simulink model "SolarPoweredPMSMDrive"  (R2024b)
settings: Solver=VariableStepAuto  StartTime=0.0  StopTime=1.5  RelTol=1e-3
libraries: spsSeriesRLCBranchLib x8, spsIGBTDiodeLib x7, spsVoltageMeasurementLib x4, spsCurrentMeasurementLib x1, spsDiodeLib x1, spsGroundLib x1, spsPVArrayLib x1, spsPWMGeneratorDCDCLib x1, simulink x1, sps_lib x1
settings Model: Creator=ASUS  LastModifiedBy=ASUS

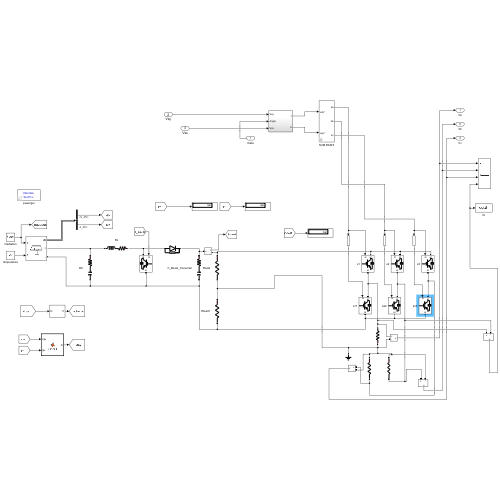
[thumbnail: Simulink's stored preview of the top-level diagram]
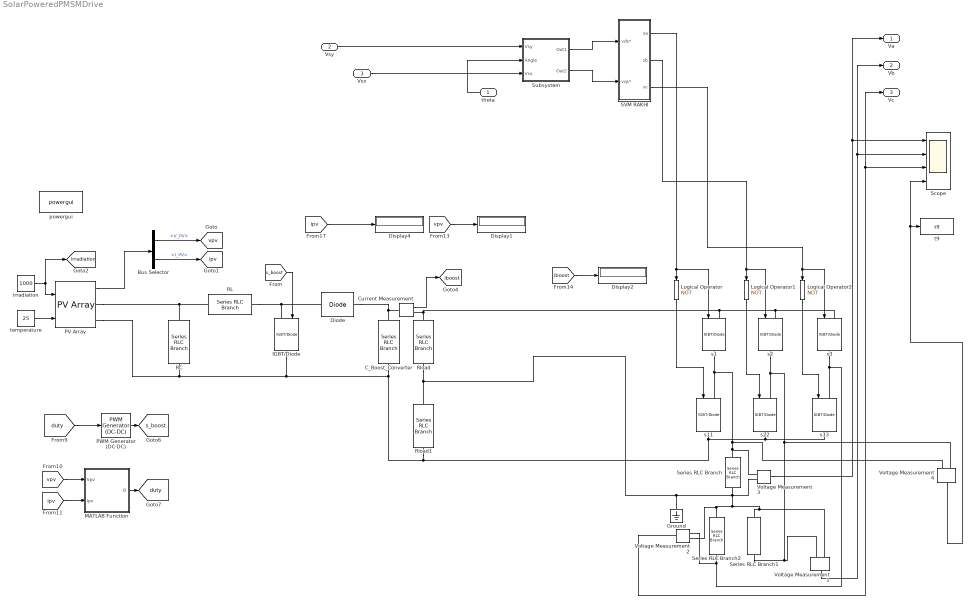
== system SolarPoweredPMSMDrive ==
  theta : Inport
  Vsy : Inport  Port=2
  Vsx : Inport  Port=3
  Bus Selector : BusSelector  OutputSignals=V_PV,I_PV
  C_Boost_Converter : spsSeriesRLCBranchLib/Series RLC Branch  LConnTagsString=__new0  RConnTagsString=__new0  BranchType=RC  Resistance=1e-4  Inductance=1e-3  SetiL0=off  InitialCurrent=0  Capacitance=660e-5  Setx0=off  InitialVoltage=0  Measurements=None
  Current Measurement : spsCurrentMeasurementLib/Current Measurement  PhasorSimulation=off  OutputType=Complex  PSBequivalent=0
  Diode : spsDiodeLib/Diode  Ron=0.001  Lon=0  Vf=0.8  IC=0  UseSnubber=0  Rs=500  Cs=250e-9  Measurements=off
  Display1 : Display
  Display2 : Display
  Display4 : Display
  Ground : spsGroundLib/Ground  LConnTagsString=a
  IGBT/Diode : spsIGBTDiodeLib/IGBT//Diode  Ron=1e-3  Rs=1e5  Cs=inf  Measurements=off
  Logical Operator : Logic  Operator=NOT  AllPortsSameDT=off  OutDataTypeStr=boolean
  Logical Operator1 : Logic  Operator=NOT  AllPortsSameDT=off  OutDataTypeStr=boolean
  Logical Operator2 : Logic  Operator=NOT  AllPortsSameDT=off  OutDataTypeStr=boolean
  MATLAB Function : MATLAB Function  TreatAsAtomicUnit=on
  PV Array : spsPVArrayLib/PV Array  Npar=10  Nser=10  PlotType=array @ 1000 W/m2 & specified temperatures  S_vec="[ 1000  500  100 ]"  Temp_C_vec="[ 45 25  ]"  ModuleName=User-defined  PlotWhenSelected=off  Pm=213.15  Ncell=60  Voc=36.3  Isc=7.84  Vm=29  Im=7.35  beta_Voc_pc=-0.36099  alpha_Isc_pc=0.102  beta_Voc=-0.13104  alpha_Isc=0.0079968  IL=7.8654  I0=2.9273e-10  nI=0.98119  Rsh=313.0553  Rs=0.39381  RobustModel=off  RobustCellTemperature=313.3991  BAL=on  Tc=1e-6  Tfilter=5e-5
  PWM Generator (DC-DC) : spsPWMGeneratorDCDCLib/PWM Generator (DC-DC)  Fsw=5000  Ts=10e-6
  RC : spsSeriesRLCBranchLib/Series RLC Branch  LConnTagsString=__new0  RConnTagsString=__new0  BranchType=RC  Resistance=1e-4  Inductance=1e-3  SetiL0=off  InitialCurrent=0  Capacitance=20e-6  Setx0=off  InitialVoltage=0  Measurements=None
  RL : spsSeriesRLCBranchLib/Series RLC Branch  LConnTagsString=__new0  RConnTagsString=__new0  BranchType=RL  Resistance=0.1  Inductance=1e-3  SetiL0=off  InitialCurrent=0  Capacitance=1e-6  Setx0=off  InitialVoltage=0  Measurements=None
  Rload : spsSeriesRLCBranchLib/Series RLC Branch  LConnTagsString=__new0  RConnTagsString=__new0  BranchType=R  Resistance=5  Inductance=1e-3  SetiL0=off  InitialCurrent=0  Capacitance=1e-6  Setx0=off  InitialVoltage=0  Measurements=None
  Rload1 : spsSeriesRLCBranchLib/Series RLC Branch  LConnTagsString=__new0  RConnTagsString=__new0  BranchType=R  Resistance=5  Inductance=1e-3  SetiL0=off  InitialCurrent=0  Capacitance=1e-6  Setx0=off  InitialVoltage=0  Measurements=None
  SVM RAKHI : Subsystem  mask{Ts=200e-6, Vdc=400}
  Scope : Scope  NumInputPorts=4
  Series RLC Branch : spsSeriesRLCBranchLib/Series RLC Branch  LConnTagsString=__new0  RConnTagsString=__new0  BranchType=R  Resistance=2  Inductance=3e-3  SetiL0=off  InitialCurrent=0  Capacitance=1e-6  Setx0=off  InitialVoltage=0  Measurements=None
  Series RLC Branch1 : spsSeriesRLCBranchLib/Series RLC Branch  LConnTagsString=__new0  RConnTagsString=__new0  BranchType=R  Resistance=2  Inductance=3e-3  SetiL0=off  InitialCurrent=0  Capacitance=1e-6  Setx0=off  InitialVoltage=0  Measurements=None
  Series RLC Branch2 : spsSeriesRLCBranchLib/Series RLC Branch  LConnTagsString=__new0  RConnTagsString=__new0  BranchType=R  Resistance=2  Inductance=3e-3  SetiL0=off  InitialCurrent=0  Capacitance=1e-6  Setx0=off  InitialVoltage=0  Measurements=None
  Subsystem : Subsystem
  Voltage Measurement{1..4} (4 alike) : spsVoltageMeasurementLib/Voltage Measurement  PhasorSimulation=off  OutputType=Complex  PSBequivalent=0
  irradiation : Constant  Value=1000
  powergui : sps_lib/powergui  Priority=1  SimulationMode=Discrete  SampleTime=50e-6  frequency=60  Iterations=50  frequencyindice=0  Pbase=100e6  ErrMax=1e-4  UnitsV=kV  UnitsW=MW  buscounter=0  FunctionMessages=off  echomessages=off  EnableUseOfTLC=off  CurrentSourceSwitches=off  DisableSnubberDevices=off  DisableRonSwitches=off  DisableVfSwitches=off  DisplayEquations=off  AutomaticDiscreteSolvers=off  SolverType=Tustin/Backward Euler (TBE)  Interpol=off  ExternalGateDelay=off  methode=off  Ts=100  x0status=blocks  SPID=on  SwTol=0  HookPort=off  NonlinearTolerance=1e-4  nMaxIteration=100  ContinueOnMaxIteration=off  RestoreLinks=warning  ResistiveCurrentMeasurement=off  Frange=[0:2:500]  Ylog=off  Xlog=on  ShowGrid=off  save=off  variable=ZData  structure=0  ZoomFFT=off  StartTime=0.0  cycles=1  DisplayStyle=1  fundamental=60  FreqAxis=off  MaxFrequency=1000  frequencyindicesteady=1  RmsSteady=1  display=off
  s{1..3,11,22,33} (6 alike) : spsIGBTDiodeLib/IGBT//Diode  Ron=1e-3  Rs=1e5  Cs=inf  Measurements=off
  t9 : ToWorkspace  VariableName=t9  SaveFormat=Structure With Time  SampleTime=-1
  temperature : Constant  Value=25
  Va : Outport
  Vb : Outport  Port=2
  Vc : Outport  Port=3
  tag scope: duty=global, iboost=global, ipv=global, irradiation=global, s_boost=global, vpv=global
  wires:
  Voltage Measurement3/1 -> Va/1, Scope/1
  Logical Operator2/1 -> s33/1
  Subsystem/1(Out1) -> SVM RAKHI/1(vds*)
  Bus Selector/1 -> [vpv]  "<V_PV>"
  irradiation/1 -> PV Array/1, [irradiation]
  [duty] -> PWM Generator (DC-DC)/1
  Bus Selector/2 -> [ipv]  "<I_PV>"
  theta/1 -> Subsystem/2(Angle)
  Voltage Measurement1/1 -> Vb/1, Scope/2
  PWM Generator (DC-DC)/1 -> [s_boost]
  [s_boost] -> IGBT/Diode/1
  [iboost] -> Display2/1
  Voltage Measurement4/1 -> t9/1, Scope/4
  [ipv] -> MATLAB Function/2(Ipv)
  SVM RAKHI/2(sb) -> Logical Operator1/1, s2/1
  [vpv] -> MATLAB Function/1(Vpv)
  Voltage Measurement2/1 -> Scope/3, Vc/1
  SVM RAKHI/3(sc) -> Logical Operator2/1, s3/1
  Vsx/1 -> Subsystem/3(Vsx)
  [vpv] -> Display1/1
  PV Array/1 -> Bus Selector/1
  Current Measurement/1 -> [iboost]
  Subsystem/2(Out2) -> SVM RAKHI/2(vqs*)
  temperature/1 -> PV Array/2
  MATLAB Function/1(D) -> [duty]
  Vsy/1 -> Subsystem/1(Vsy)
  [ipv] -> Display4/1
  Logical Operator/1 -> s11/1
  Logical Operator1/1 -> s22/1
  SVM RAKHI/1(sa) -> Logical Operator/1, s1/1
  connections:
  Diode/RConn1 -- Current Measurement/LConn1 -- C_Boost_Converter/LConn1
  Series RLC Branch1/RConn1 -- Voltage Measurement1/LConn1 -- s22/LConn1 -- s2/RConn1 -- Voltage Measurement4/LConn2
  PV Array/RConn1 -- RL/RConn1 -- RC/LConn1
  s1/RConn1 -- Voltage Measurement3/LConn1 -- Series RLC Branch/RConn1 -- Voltage Measurement4/LConn1 -- s11/LConn1
  s3/RConn1 -- Voltage Measurement2/LConn1 -- Series RLC Branch2/RConn1 -- s33/LConn1
  s22/RConn1 -- s33/RConn1 -- s11/RConn1 -- Rload1/RConn1 -- C_Boost_Converter/RConn1 -- IGBT/Diode/RConn1 -- PV Array/RConn2 -- RC/RConn1
  Voltage Measurement2/LConn2 -- Series RLC Branch2/LConn1 -- Series RLC Branch1/LConn1 -- Voltage Measurement1/LConn2 -- Voltage Measurement3/LConn2 -- Ground/LConn1 -- Rload1/LConn1 -- Rload/RConn1 -- Series RLC Branch/LConn1
  s2/LConn1 -- Rload/LConn1 -- Current Measurement/RConn1 -- s1/LConn1 -- s3/LConn1
  Diode/LConn1 -- RL/LConn1 -- IGBT/Diode/LConn1

== system SolarPoweredPMSMDrive/SVM RAKHI ==
  vds* : Inport
  vqs* : Inport  Port=2
  Angle Estimator : Subsystem  mask(angle estimator){}
  twolevel svm1rakhi : Subsystem
  sa : Outport
  sb : Outport  Port=2
  sc : Outport  Port=3
  wires:
  vqs*/1 -> Angle Estimator/2(vqs*)
  vds*/1 -> Angle Estimator/1(vds*)
  Angle Estimator/1(alpha) -> twolevel svm1rakhi/1(alpha)
  Angle Estimator/2(vref) -> twolevel svm1rakhi/2(VS)
  twolevel svm1rakhi/1(Sa) -> sa/1
  twolevel svm1rakhi/2(Sb) -> sb/1
  twolevel svm1rakhi/3(Sc) -> sc/1

== system SolarPoweredPMSMDrive/Subsystem ==
  Vsy : Inport
  Angle : Inport  Port=2
  Vsx : Inport  Port=3
  Mux1 : Mux  Inputs=3
      settings: DisplayOption=signals
  Vds : Fcn  Expr=(cos(u(3))*u(1))-(sin(u(3))*u(2))
  Vqs : Fcn  Expr=(cos(u(3))*u(2))+(sin(u(3))*u(1))
  Out1 : Outport
  Out2 : Outport  Port=2
  wires:
  Vds/1 -> Out1/1
  Vsy/1 -> Mux1/2
  Vsx/1 -> Mux1/1
  Angle/1 -> Mux1/3
  Vqs/1 -> Out2/1
  Mux1/1 -> Vds/1, Vqs/1

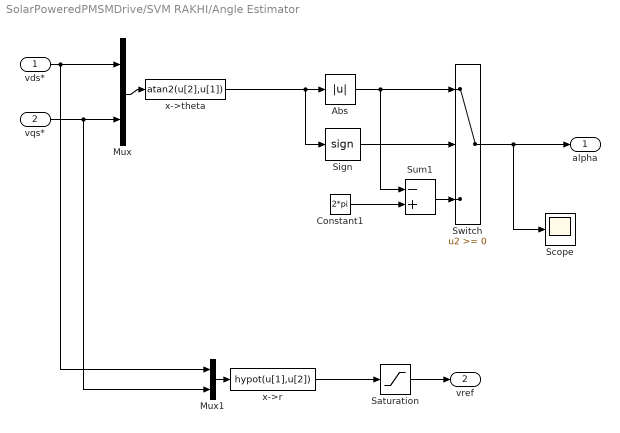
== system SolarPoweredPMSMDrive/SVM RAKHI/Angle Estimator ==
  vds* : Inport
  vqs* : Inport  Port=2
  Abs : Abs
  Constant1 : Constant  Value=2*pi
  Mux : Mux  Inputs=2
  Mux1 : Mux  Inputs=2
  Saturation : Saturate  UpperLimit=Vdc/1.732  LowerLimit=0
  Scope : Scope
  Sign : Signum
  Sum1 : Sum  Inputs=-+  InputSameDT=on  SaturateOnIntegerOverflow=on  OutDataTypeStr=Inherit: Same as first input
  Switch : Switch
  x->r : Fcn  Expr=hypot(u[1],u[2])
  x->theta : Fcn  Expr=atan2(u[2],u[1])
  alpha : Outport
  vref : Outport  Port=2
  wires:
  Abs/1 -> Sum1/1, Switch/1
  Sign/1 -> Switch/2
  Constant1/1 -> Sum1/2
  Sum1/1 -> Switch/3
  Switch/1 -> Scope/1, alpha/1
  x->theta/1 -> Sign/1, Abs/1
  Mux/1 -> x->theta/1
  x->r/1 -> Saturation/1
  vqs*/1 -> Mux/2, Mux1/2
  vds*/1 -> Mux/1, Mux1/1
  Mux1/1 -> x->r/1
  Saturation/1 -> vref/1

== system SolarPoweredPMSMDrive/SVM RAKHI/twolevel svm1rakhi ==
  alpha : Inport
  VS : Inport  Port=2
  Repeating Sequence : simulink/Sources/Repeating Sequence  rep_seq_t=[0 200e-6]  rep_seq_y=[0 200e-6]
  Subsystem2 : Subsystem
  Subsystem3 : Subsystem  mask{Ts=200e-6, Vdc=530}
  final two level pulses : Subsystem
  Sa : Outport
  Sb : Outport  Port=2
  Sc : Outport  Port=3
  wires:
  Subsystem3/2(Tb) -> final two level pulses/4(Tb)
  Subsystem3/3(T0) -> final two level pulses/5(T0)
  Repeating Sequence/1 -> final two level pulses/2(Cr)
  Subsystem3/1(Ta) -> final two level pulses/3(Ta)
  Subsystem2/1(K) -> Subsystem3/1(K), final two level pulses/1(K)
  alpha/1 -> Subsystem2/1(alpha), Subsystem3/2(ALPHA)
  VS/1 -> Subsystem3/3(VS)
  final two level pulses/2(Sb) -> Sb/1
  final two level pulses/1(Sa) -> Sa/1
  final two level pulses/3(Sc) -> Sc/1

== system SolarPoweredPMSMDrive/SVM RAKHI/twolevel svm1rakhi/Subsystem2 ==
  alpha : Inport
  Display : Display
  Fcn : Fcn  Expr=(3*u/pi)+1
  Rounding Function : Rounding  Operator=fix
  K : Outport
  wires:
  Fcn/1 -> Rounding Function/1
  alpha/1 -> Fcn/1
  Rounding Function/1 -> K/1, Display/1

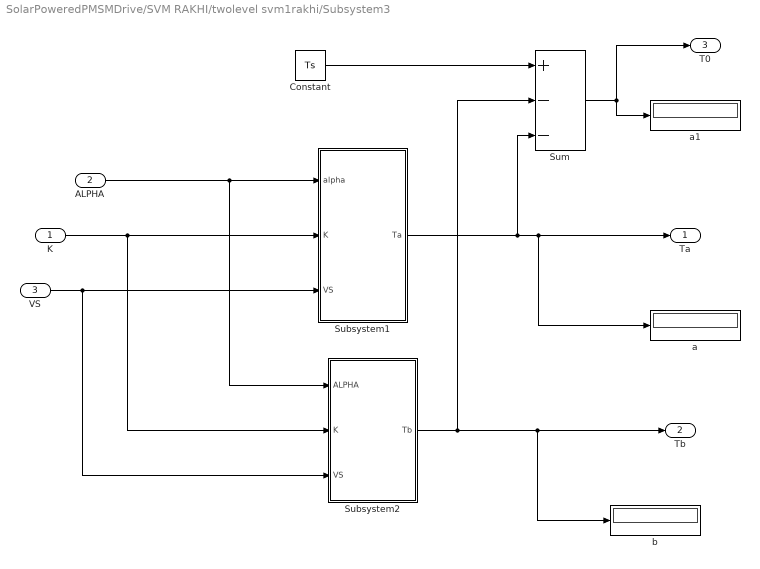
== system SolarPoweredPMSMDrive/SVM RAKHI/twolevel svm1rakhi/Subsystem3 ==
  K : Inport
  ALPHA : Inport  Port=2
  VS : Inport  Port=3
  Constant : Constant  Value=Ts
  Subsystem1 : Subsystem
  Subsystem2 : Subsystem
  Sum : Sum  Inputs=+--
  a : Display
  a1 : Display
  b : Display
  Ta : Outport
  Tb : Outport  Port=2
  T0 : Outport  Port=3
  wires:
  Sum/1 -> a1/1, T0/1
  Constant/1 -> Sum/1
  Subsystem2/1(Tb) -> b/1, Tb/1, Sum/2
  K/1 -> Subsystem2/2(K), Subsystem1/2(K)
  Subsystem1/1(Ta) -> a/1, Ta/1, Sum/3
  ALPHA/1 -> Subsystem1/1(alpha), Subsystem2/1(ALPHA)
  VS/1 -> Subsystem1/3(VS), Subsystem2/3(VS)

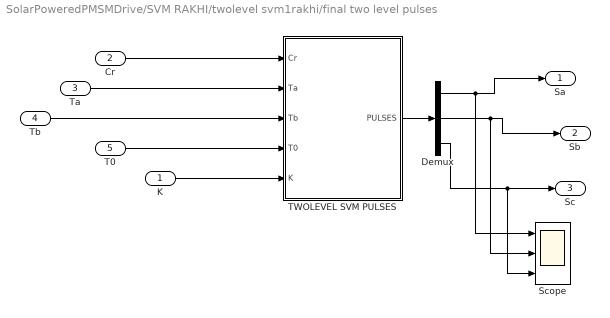
== system SolarPoweredPMSMDrive/SVM RAKHI/twolevel svm1rakhi/final two level pulses ==
  K : Inport
  Cr : Inport  Port=2
  Ta : Inport  Port=3
  Tb : Inport  Port=4
  T0 : Inport  Port=5
  Demux : Demux  Outputs=3
  Scope : Scope  NumInputPorts=3
  TWOLEVEL SVM PULSES : Subsystem
  Sa : Outport
  Sb : Outport  Port=2
  Sc : Outport  Port=3
  wires:
  TWOLEVEL SVM PULSES/1(PULSES) -> Demux/1
  Cr/1 -> TWOLEVEL SVM PULSES/1(Cr)
  Ta/1 -> TWOLEVEL SVM PULSES/2(Ta)
  Demux/3 -> Sc/1, Scope/3
  T0/1 -> TWOLEVEL SVM PULSES/4(T0)
  Demux/1 -> Sa/1, Scope/1
  Tb/1 -> TWOLEVEL SVM PULSES/3(Tb)
  Demux/2 -> Sb/1, Scope/2
  K/1 -> TWOLEVEL SVM PULSES/5(K)

== system SolarPoweredPMSMDrive/SVM RAKHI/twolevel svm1rakhi/Subsystem3/Subsystem1 ==
  alpha : Inport
  K : Inport  Port=2
  VS : Inport  Port=3
  Display : Display
  Fcn : Fcn  Expr=sin(u)
  Gain : Gain  Gain=pi/3
  Gain1 : Gain  Gain=(Ts/Vdc)*1.732
  Product1 : Product
  Sum : Sum  Inputs=-+
  Ta : Outport
  wires:
  alpha/1 -> Sum/1
  Product1/1 -> Ta/1, Display/1
  Sum/1 -> Fcn/1
  Gain/1 -> Sum/2
  Fcn/1 -> Gain1/1
  Gain1/1 -> Product1/1
  K/1 -> Gain/1
  VS/1 -> Product1/2

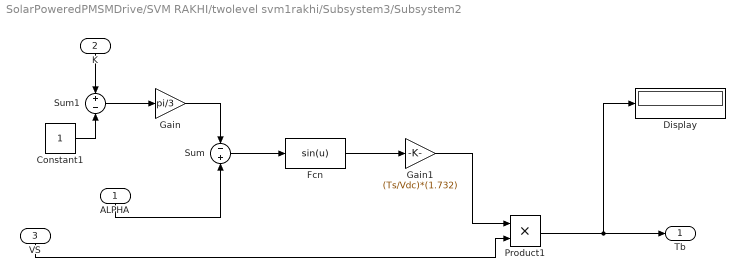
== system SolarPoweredPMSMDrive/SVM RAKHI/twolevel svm1rakhi/Subsystem3/Subsystem2 ==
  ALPHA : Inport
  K : Inport  Port=2
  VS : Inport  Port=3
  Constant1 : Constant
  Display : Display
  Fcn : Fcn  Expr=sin(u)
  Gain : Gain  Gain=pi/3
  Gain1 : Gain  Gain=(Ts/Vdc)*(1.732)
  Product1 : Product
  Sum : Sum  Inputs=-+
  Sum1 : Sum  Inputs=+-
  Tb : Outport
  wires:
  Sum/1 -> Fcn/1
  Fcn/1 -> Gain1/1
  Gain/1 -> Sum/1
  Gain1/1 -> Product1/1
  K/1 -> Sum1/1
  ALPHA/1 -> Sum/2
  VS/1 -> Product1/2
  Constant1/1 -> Sum1/2
  Product1/1 -> Tb/1, Display/1
  Sum1/1 -> Gain/1

== system SolarPoweredPMSMDrive/SVM RAKHI/twolevel svm1rakhi/final two level pulses/TWOLEVEL SVM PULSES ==
  Cr : Inport
  Ta : Inport  Port=2
  Tb : Inport  Port=3
  T0 : Inport  Port=4
  K : Inport  Port=5
  Multiport Switch : MultiPortSwitch  Inputs=6  DiagnosticForDefault=None  SaturateOnIntegerOverflow=off  InputSameDT=off
  PULSES FOR ALL SECTORS : Subsystem
  PULSES : Outport
  wires:
  K/1 -> Multiport Switch/1
  Ta/1 -> PULSES FOR ALL SECTORS/2(Ta)
  Tb/1 -> PULSES FOR ALL SECTORS/3(Tb)
  T0/1 -> PULSES FOR ALL SECTORS/4(T0)
  PULSES FOR ALL SECTORS/2(sector2) -> Multiport Switch/3
  PULSES FOR ALL SECTORS/1(sector1) -> Multiport Switch/2
  PULSES FOR ALL SECTORS/5(sector5) -> Multiport Switch/6
  PULSES FOR ALL SECTORS/4(sector4) -> Multiport Switch/5
  PULSES FOR ALL SECTORS/3(sector3) -> Multiport Switch/4
  PULSES FOR ALL SECTORS/6(sector6) -> Multiport Switch/7
  Cr/1 -> PULSES FOR ALL SECTORS/1(Cr)
  Multiport Switch/1 -> PULSES/1

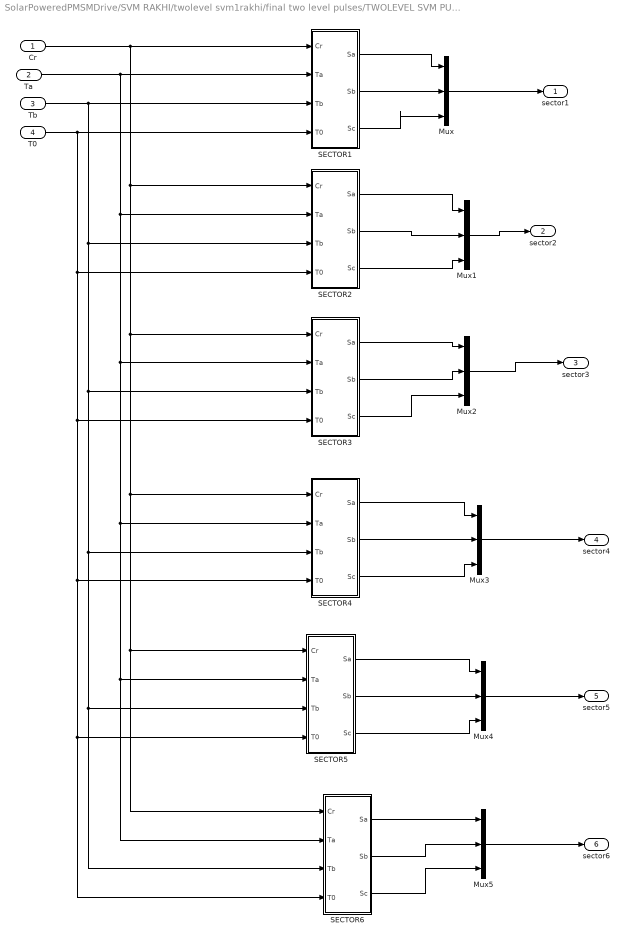
== system SolarPoweredPMSMDrive/SVM RAKHI/twolevel svm1rakhi/final two level pulses/TWOLEVEL SVM PULSES/PULSES FOR ALL SECTORS ==
  Cr : Inport
  Ta : Inport  Port=2
  Tb : Inport  Port=3
  T0 : Inport  Port=4
  Mux{,1..5} (6 alike) : Mux  Inputs=3
  SECTOR1 : Subsystem
  SECTOR2 : Subsystem
  SECTOR3 : Subsystem
  SECTOR4 : Subsystem
  SECTOR5 : Subsystem
  SECTOR6 : Subsystem
  sector1 : Outport
  sector2 : Outport  Port=2
  sector3 : Outport  Port=3
  sector4 : Outport  Port=4
  sector5 : Outport  Port=5
  sector6 : Outport  Port=6
  wires:
  SECTOR6/3(Sc) -> Mux5/3
  Mux4/1 -> sector5/1
  Mux/1 -> sector1/1
  Mux5/1 -> sector6/1
  Mux3/1 -> sector4/1
  SECTOR6/2(Sb) -> Mux5/2
  SECTOR5/3(Sc) -> Mux4/3
  Mux1/1 -> sector2/1
  SECTOR5/2(Sb) -> Mux4/2
  Mux2/1 -> sector3/1
  SECTOR3/2(Sb) -> Mux2/2
  SECTOR1/1(Sa) -> Mux/1
  SECTOR1/2(Sb) -> Mux/2
  SECTOR4/2(Sb) -> Mux3/2
  SECTOR4/3(Sc) -> Mux3/3
  SECTOR2/1(Sa) -> Mux1/1
  SECTOR6/1(Sa) -> Mux5/1
  SECTOR1/3(Sc) -> Mux/3
  SECTOR3/1(Sa) -> Mux2/1
  SECTOR4/1(Sa) -> Mux3/1
  SECTOR3/3(Sc) -> Mux2/3
  SECTOR5/1(Sa) -> Mux4/1
  SECTOR2/3(Sc) -> Mux1/3
  SECTOR2/2(Sb) -> Mux1/2
  Cr/1 -> SECTOR1/1(Cr), SECTOR2/1(Cr), SECTOR4/1(Cr), SECTOR6/1(Cr), SECTOR5/1(Cr), SECTOR3/1(Cr)
  T0/1 -> SECTOR6/4(T0), SECTOR5/4(T0), SECTOR4/4(T0), SECTOR3/4(T0), SECTOR2/4(T0), SECTOR1/4(T0)
  Ta/1 -> SECTOR1/2(Ta), SECTOR3/2(Ta), SECTOR4/2(Ta), SECTOR6/2(Ta), SECTOR5/2(Ta), SECTOR2/2(Ta)
  Tb/1 -> SECTOR1/3(Tb), SECTOR5/3(Tb), SECTOR6/3(Tb), SECTOR4/3(Tb), SECTOR3/3(Tb), SECTOR2/3(Tb)

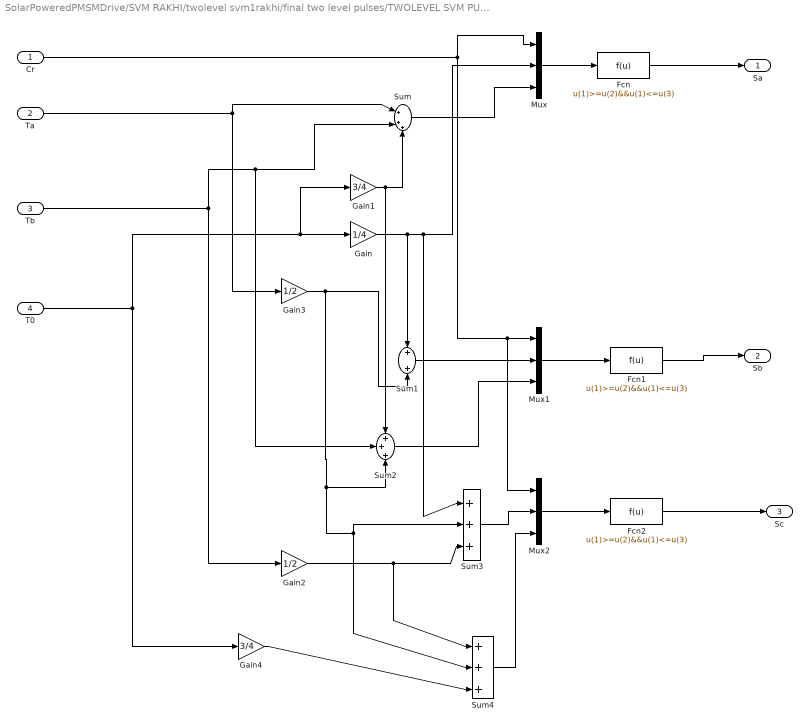
== system SolarPoweredPMSMDrive/SVM RAKHI/twolevel svm1rakhi/final two level pulses/TWOLEVEL SVM PULSES/PULSES FOR ALL SECTORS/SECTOR1 ==
  Cr : Inport
  Ta : Inport  Port=2
  Tb : Inport  Port=3
  T0 : Inport  Port=4
  Fcn : Fcn  Expr=u(1)>=u(2)&&u(1)<=u(3)
  Fcn1 : Fcn  Expr=u(1)>=u(2)&&u(1)<=u(3)
  Fcn2 : Fcn  Expr=u(1)>=u(2)&&u(1)<=u(3)
  Gain : Gain  Gain=1/4
  Gain1 : Gain  Gain=3/4
  Gain2 : Gain  Gain=1/2
  Gain3 : Gain  Gain=1/2
  Gain4 : Gain  Gain=3/4
  Mux : Mux  Inputs=3
  Mux1 : Mux  Inputs=3
  Mux2 : Mux  Inputs=3
  Sum : Sum  Inputs=|+++
  Sum1 : Sum
  Sum2 : Sum  Inputs=+++
  Sum3 : Sum  Inputs=|+++
  Sum4 : Sum  Inputs=|+++
  Sa : Outport
  Sb : Outport  Port=2
  Sc : Outport  Port=3
  wires:
  Sum2/1 -> Mux1/3
  Mux/1 -> Fcn/1
  T0/1 -> Gain4/1, Gain1/1, Gain/1
  Sum1/1 -> Mux1/2
  Mux2/1 -> Fcn2/1
  Gain3/1 -> Sum4/2, Sum3/2, Sum2/3, Sum1/2
  Gain1/1 -> Sum/3, Sum2/1
  Sum/1 -> Mux/3
  Fcn2/1 -> Sc/1
  Sum4/1 -> Mux2/3
  Cr/1 -> Mux/1, Mux2/1, Mux1/1
  Fcn/1 -> Sa/1
  Gain2/1 -> Sum4/1, Sum3/3
  Mux1/1 -> Fcn1/1
  Sum3/1 -> Mux2/2
  Gain4/1 -> Sum4/3
  Fcn1/1 -> Sb/1
  Gain/1 -> Sum3/1, Mux/2, Sum1/1
  Ta/1 -> Gain3/1, Sum/1
  Tb/1 -> Sum2/2, Sum/2, Gain2/1

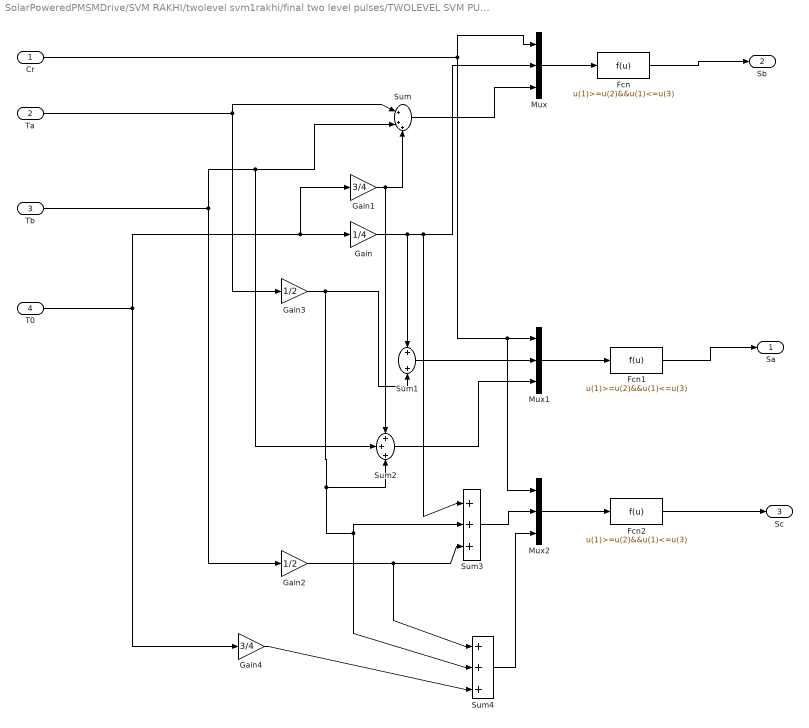
== system SolarPoweredPMSMDrive/SVM RAKHI/twolevel svm1rakhi/final two level pulses/TWOLEVEL SVM PULSES/PULSES FOR ALL SECTORS/SECTOR2 ==
  Cr : Inport
  Ta : Inport  Port=2
  Tb : Inport  Port=3
  T0 : Inport  Port=4
  Fcn : Fcn  Expr=u(1)>=u(2)&&u(1)<=u(3)
  Fcn1 : Fcn  Expr=u(1)>=u(2)&&u(1)<=u(3)
  Fcn2 : Fcn  Expr=u(1)>=u(2)&&u(1)<=u(3)
  Gain : Gain  Gain=1/4
  Gain1 : Gain  Gain=3/4
  Gain2 : Gain  Gain=1/2
  Gain3 : Gain  Gain=1/2
  Gain4 : Gain  Gain=3/4
  Mux : Mux  Inputs=3
  Mux1 : Mux  Inputs=3
  Mux2 : Mux  Inputs=3
  Sum : Sum  Inputs=|+++
  Sum1 : Sum
  Sum2 : Sum  Inputs=+++
  Sum3 : Sum  Inputs=|+++
  Sum4 : Sum  Inputs=|+++
  Sa : Outport
  Sb : Outport  Port=2
  Sc : Outport  Port=3
  wires:
  Fcn2/1 -> Sc/1
  Fcn/1 -> Sb/1
  Fcn1/1 -> Sa/1
  Tb/1 -> Gain2/1, Sum/2, Sum2/2
  Ta/1 -> Sum/1, Gain3/1
  Gain/1 -> Sum1/1, Mux/2, Sum3/1
  Gain4/1 -> Sum4/3
  Sum3/1 -> Mux2/2
  Mux1/1 -> Fcn1/1
  Gain2/1 -> Sum3/3, Sum4/1
  Cr/1 -> Mux1/1, Mux2/1, Mux/1
  Sum4/1 -> Mux2/3
  Sum/1 -> Mux/3
  Gain1/1 -> Sum2/1, Sum/3
  Gain3/1 -> Sum1/2, Sum2/3, Sum3/2, Sum4/2
  Mux2/1 -> Fcn2/1
  Sum1/1 -> Mux1/2
  T0/1 -> Gain/1, Gain1/1, Gain4/1
  Mux/1 -> Fcn/1
  Sum2/1 -> Mux1/3

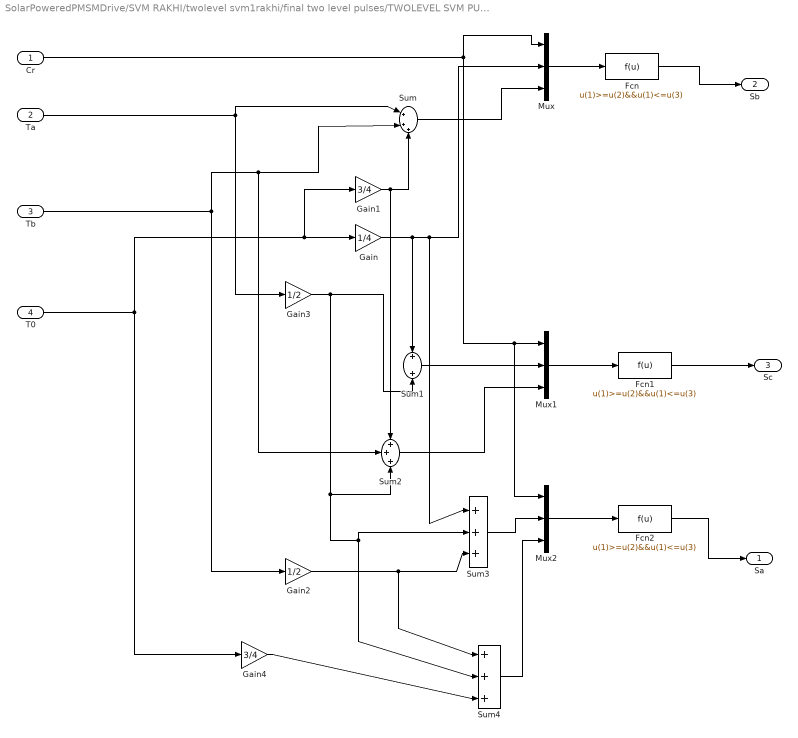
== system SolarPoweredPMSMDrive/SVM RAKHI/twolevel svm1rakhi/final two level pulses/TWOLEVEL SVM PULSES/PULSES FOR ALL SECTORS/SECTOR3 ==
  Cr : Inport
  Ta : Inport  Port=2
  Tb : Inport  Port=3
  T0 : Inport  Port=4
  Fcn : Fcn  Expr=u(1)>=u(2)&&u(1)<=u(3)
  Fcn1 : Fcn  Expr=u(1)>=u(2)&&u(1)<=u(3)
  Fcn2 : Fcn  Expr=u(1)>=u(2)&&u(1)<=u(3)
  Gain : Gain  Gain=1/4
  Gain1 : Gain  Gain=3/4
  Gain2 : Gain  Gain=1/2
  Gain3 : Gain  Gain=1/2
  Gain4 : Gain  Gain=3/4
  Mux : Mux  Inputs=3
  Mux1 : Mux  Inputs=3
  Mux2 : Mux  Inputs=3
  Sum : Sum  Inputs=|+++
  Sum1 : Sum
  Sum2 : Sum  Inputs=+++
  Sum3 : Sum  Inputs=|+++
  Sum4 : Sum  Inputs=|+++
  Sa : Outport
  Sb : Outport  Port=2
  Sc : Outport  Port=3
  wires:
  Fcn1/1 -> Sc/1
  Fcn/1 -> Sb/1
  Fcn2/1 -> Sa/1
  Tb/1 -> Gain2/1, Sum/2, Sum2/2
  Ta/1 -> Sum/1, Gain3/1
  Gain/1 -> Sum1/1, Mux/2, Sum3/1
  Gain4/1 -> Sum4/3
  Sum3/1 -> Mux2/2
  Mux1/1 -> Fcn1/1
  Gain2/1 -> Sum3/3, Sum4/1
  Cr/1 -> Mux1/1, Mux2/1, Mux/1
  Sum4/1 -> Mux2/3
  Sum/1 -> Mux/3
  Gain1/1 -> Sum2/1, Sum/3
  Gain3/1 -> Sum1/2, Sum2/3, Sum3/2, Sum4/2
  Mux2/1 -> Fcn2/1
  Sum1/1 -> Mux1/2
  T0/1 -> Gain/1, Gain1/1, Gain4/1
  Mux/1 -> Fcn/1
  Sum2/1 -> Mux1/3

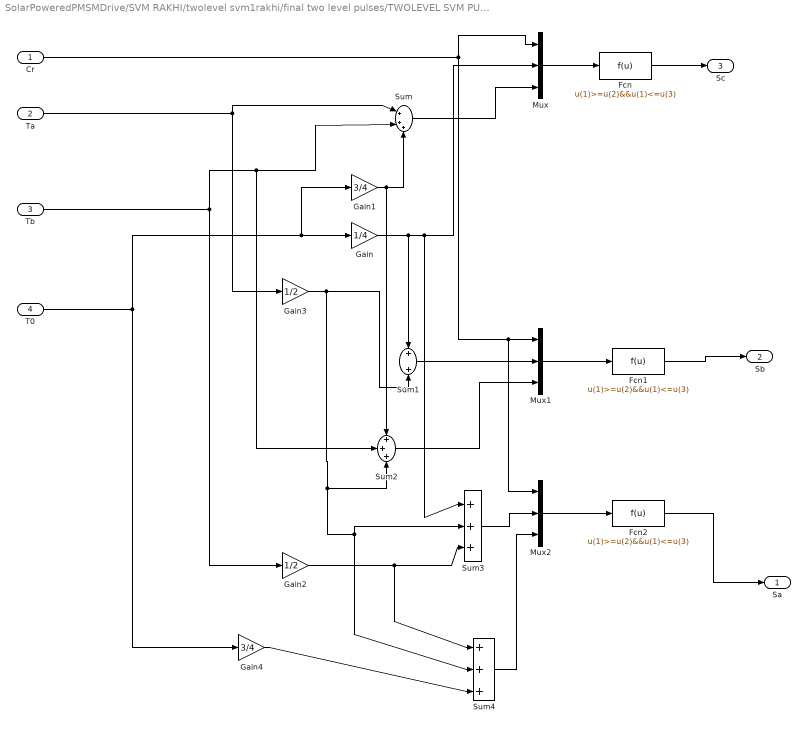
== system SolarPoweredPMSMDrive/SVM RAKHI/twolevel svm1rakhi/final two level pulses/TWOLEVEL SVM PULSES/PULSES FOR ALL SECTORS/SECTOR4 ==
  Cr : Inport
  Ta : Inport  Port=2
  Tb : Inport  Port=3
  T0 : Inport  Port=4
  Fcn : Fcn  Expr=u(1)>=u(2)&&u(1)<=u(3)
  Fcn1 : Fcn  Expr=u(1)>=u(2)&&u(1)<=u(3)
  Fcn2 : Fcn  Expr=u(1)>=u(2)&&u(1)<=u(3)
  Gain : Gain  Gain=1/4
  Gain1 : Gain  Gain=3/4
  Gain2 : Gain  Gain=1/2
  Gain3 : Gain  Gain=1/2
  Gain4 : Gain  Gain=3/4
  Mux : Mux  Inputs=3
  Mux1 : Mux  Inputs=3
  Mux2 : Mux  Inputs=3
  Sum : Sum  Inputs=|+++
  Sum1 : Sum
  Sum2 : Sum  Inputs=+++
  Sum3 : Sum  Inputs=|+++
  Sum4 : Sum  Inputs=|+++
  Sa : Outport
  Sb : Outport  Port=2
  Sc : Outport  Port=3
  wires:
  Fcn/1 -> Sc/1
  Fcn1/1 -> Sb/1
  Fcn2/1 -> Sa/1
  Tb/1 -> Gain2/1, Sum/2, Sum2/2
  Ta/1 -> Sum/1, Gain3/1
  Gain/1 -> Sum1/1, Mux/2, Sum3/1
  Gain4/1 -> Sum4/3
  Sum3/1 -> Mux2/2
  Mux1/1 -> Fcn1/1
  Gain2/1 -> Sum3/3, Sum4/1
  Cr/1 -> Mux1/1, Mux2/1, Mux/1
  Sum4/1 -> Mux2/3
  Sum/1 -> Mux/3
  Gain1/1 -> Sum2/1, Sum/3
  Gain3/1 -> Sum1/2, Sum2/3, Sum3/2, Sum4/2
  Mux2/1 -> Fcn2/1
  Sum1/1 -> Mux1/2
  T0/1 -> Gain/1, Gain1/1, Gain4/1
  Mux/1 -> Fcn/1
  Sum2/1 -> Mux1/3

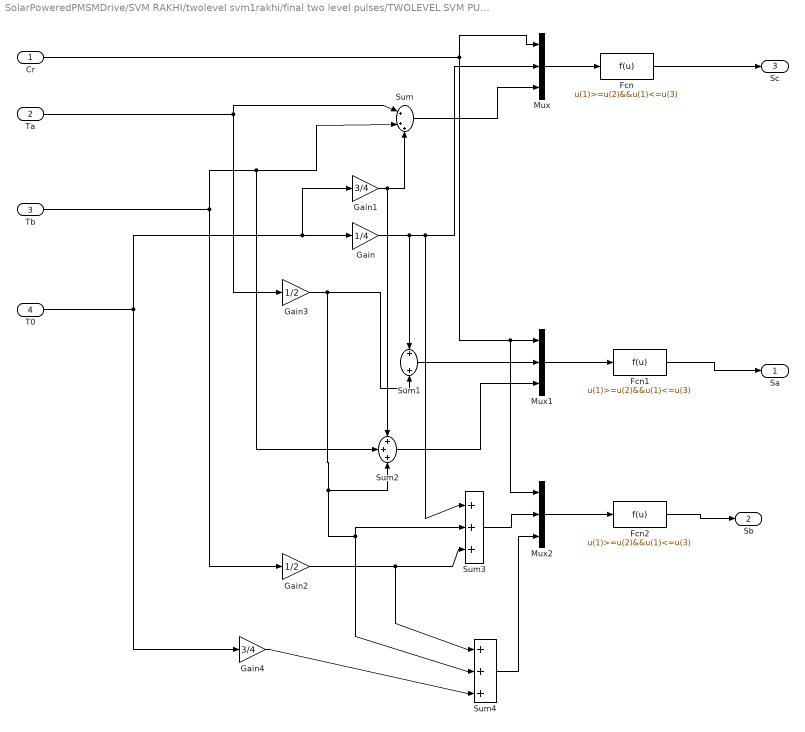
== system SolarPoweredPMSMDrive/SVM RAKHI/twolevel svm1rakhi/final two level pulses/TWOLEVEL SVM PULSES/PULSES FOR ALL SECTORS/SECTOR5 ==
  Cr : Inport
  Ta : Inport  Port=2
  Tb : Inport  Port=3
  T0 : Inport  Port=4
  Fcn : Fcn  Expr=u(1)>=u(2)&&u(1)<=u(3)
  Fcn1 : Fcn  Expr=u(1)>=u(2)&&u(1)<=u(3)
  Fcn2 : Fcn  Expr=u(1)>=u(2)&&u(1)<=u(3)
  Gain : Gain  Gain=1/4
  Gain1 : Gain  Gain=3/4
  Gain2 : Gain  Gain=1/2
  Gain3 : Gain  Gain=1/2
  Gain4 : Gain  Gain=3/4
  Mux : Mux  Inputs=3
  Mux1 : Mux  Inputs=3
  Mux2 : Mux  Inputs=3
  Sum : Sum  Inputs=|+++
  Sum1 : Sum
  Sum2 : Sum  Inputs=+++
  Sum3 : Sum  Inputs=|+++
  Sum4 : Sum  Inputs=|+++
  Sa : Outport
  Sb : Outport  Port=2
  Sc : Outport  Port=3
  wires:
  Fcn/1 -> Sc/1
  Fcn2/1 -> Sb/1
  Fcn1/1 -> Sa/1
  Tb/1 -> Gain2/1, Sum/2, Sum2/2
  Ta/1 -> Sum/1, Gain3/1
  Gain/1 -> Sum1/1, Mux/2, Sum3/1
  Gain4/1 -> Sum4/3
  Sum3/1 -> Mux2/2
  Mux1/1 -> Fcn1/1
  Gain2/1 -> Sum3/3, Sum4/1
  Cr/1 -> Mux1/1, Mux2/1, Mux/1
  Sum4/1 -> Mux2/3
  Sum/1 -> Mux/3
  Gain1/1 -> Sum2/1, Sum/3
  Gain3/1 -> Sum1/2, Sum2/3, Sum3/2, Sum4/2
  Mux2/1 -> Fcn2/1
  Sum1/1 -> Mux1/2
  T0/1 -> Gain/1, Gain1/1, Gain4/1
  Mux/1 -> Fcn/1
  Sum2/1 -> Mux1/3

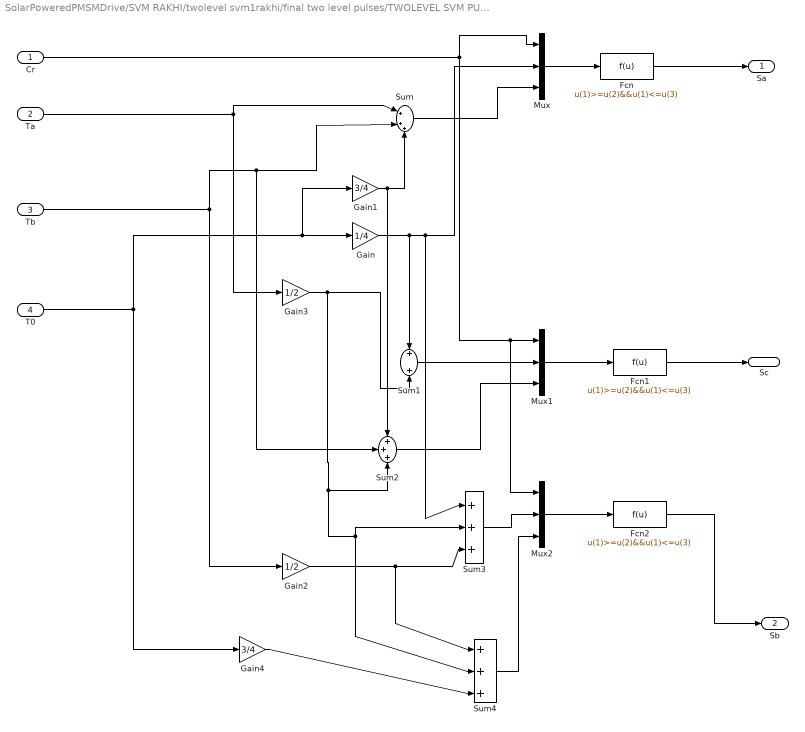
== system SolarPoweredPMSMDrive/SVM RAKHI/twolevel svm1rakhi/final two level pulses/TWOLEVEL SVM PULSES/PULSES FOR ALL SECTORS/SECTOR6 ==
  Cr : Inport
  Ta : Inport  Port=2
  Tb : Inport  Port=3
  T0 : Inport  Port=4
  Fcn : Fcn  Expr=u(1)>=u(2)&&u(1)<=u(3)
  Fcn1 : Fcn  Expr=u(1)>=u(2)&&u(1)<=u(3)
  Fcn2 : Fcn  Expr=u(1)>=u(2)&&u(1)<=u(3)
  Gain : Gain  Gain=1/4
  Gain1 : Gain  Gain=3/4
  Gain2 : Gain  Gain=1/2
  Gain3 : Gain  Gain=1/2
  Gain4 : Gain  Gain=3/4
  Mux : Mux  Inputs=3
  Mux1 : Mux  Inputs=3
  Mux2 : Mux  Inputs=3
  Sum : Sum  Inputs=|+++
  Sum1 : Sum
  Sum2 : Sum  Inputs=+++
  Sum3 : Sum  Inputs=|+++
  Sum4 : Sum  Inputs=|+++
  Sa : Outport
  Sb : Outport  Port=2
  Sc : Outport  Port=3
  wires:
  Fcn/1 -> Sa/1
  Fcn1/1 -> Sc/1
  Fcn2/1 -> Sb/1
  Tb/1 -> Gain2/1, Sum/2, Sum2/2
  Ta/1 -> Sum/1, Gain3/1
  Gain/1 -> Sum1/1, Mux/2, Sum3/1
  Gain4/1 -> Sum4/3
  Sum3/1 -> Mux2/2
  Mux1/1 -> Fcn1/1
  Gain2/1 -> Sum3/3, Sum4/1
  Cr/1 -> Mux1/1, Mux2/1, Mux/1
  Sum4/1 -> Mux2/3
  Sum/1 -> Mux/3
  Gain1/1 -> Sum2/1, Sum/3
  Gain3/1 -> Sum1/2, Sum2/3, Sum3/2, Sum4/2
  Mux2/1 -> Fcn2/1
  Sum1/1 -> Mux1/2
  T0/1 -> Gain/1, Gain1/1, Gain4/1
  Mux/1 -> Fcn/1
  Sum2/1 -> Mux1/3

== matlab function SolarPoweredPMSMDrive/MATLAB Function ==
  data: Vpv input; D output; Ipv input
function D= PandO(Vpv,Ipv)
persistent Dprev Pprev Vprev
if isempty(Dprev)
    Dprev=0.7;
    Vprev=29;
    Pprev=213.15;
end

deltaD=125e-6;
%calculate measured array power
Ppv=Vpv*Ipv;
%Increase or decrease duty cycle based on conditions
if(Ppv-Pprev)~=0
    if(Ppv-Pprev)>0
       if (Vpv-Vprev)>0
           D=Dprev-deltaD;
       else
           D=Dprev+deltaD;
       end
    else
        if(Vpv-Vprev)>0
            D=Dprev+deltaD;
        else
            D=Dprev-deltaD;
        end
    end
else
    D=Dprev;
end
%Update internal valules
Dprev=D;
Vprev=Vpv;
Pprev=Ppv;
